simulink model "Ejemplo_3"  (R2013a)
settings: Solver=ode45  StartTime=0.0  StopTime=10.0  RelTol=1e-3
settings Model: Creator=Miguel  LastModifiedBy=Miguel

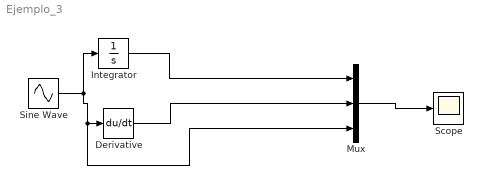
== system Ejemplo_3 ==
  Derivative : Derivative
  Integrator : Integrator  InitialCondition=-1
  Mux : Mux  Inputs=3
  Scope : Scope
      settings: ShowLegends=on
  Sine Wave : Sin  SampleTime=0
  wires:
  Sine Wave/1 -> Integrator/1, Mux/3, Derivative/1
  Integrator/1 -> Mux/1
  Derivative/1 -> Mux/2
  Mux/1 -> Scope/1
